simulink model "reference_model"  (R2023a)
settings: Solver=VariableStepAuto  StartTime=0.0  StopTime=200  RelTol=1e-3
values from neighbouring files (symbols this model uses):
  Af = diag ([1/t1, 1/t2, 1/t3])    [init.m]
  Gamma_Matrix = diag(omega.^2)    [init.m]
  Omega_Matrix = diag (2*zeta.*omega)    [init.m]
libraries: eeStairGenerator x3
settings Model: Creator=33769  LastModifiedBy=33769

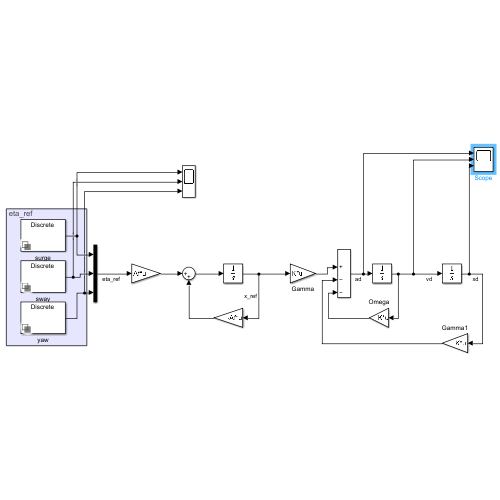
[thumbnail: Simulink's stored preview of the top-level diagram]
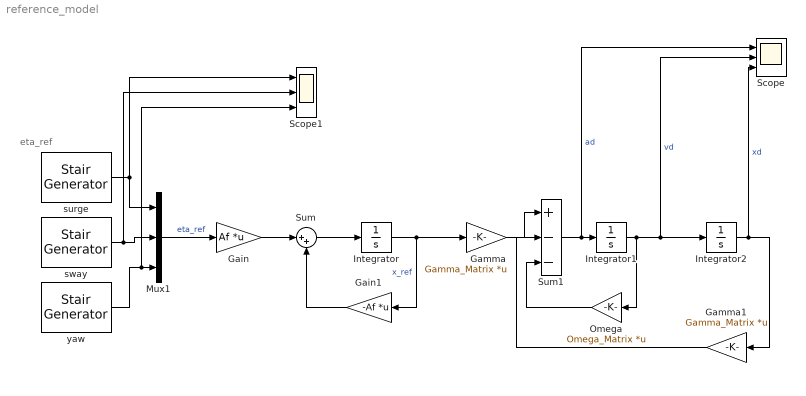
== system reference_model ==
  note: eta_ref
  Gain : Gain  Gain=Af  Multiplication=Matrix(K*u)
  Gain1 : Gain  Gain=-Af  Multiplication=Matrix(K*u)
  Gamma : Gain  Gain=Gamma_Matrix  Multiplication=Matrix(K*u)
  Gamma1 : Gain  Gain=Gamma_Matrix  Multiplication=Matrix(K*u)
  Integrator : Integrator
  Integrator1 : Integrator
  Integrator2 : Integrator
  Mux1 : Mux  Inputs=3
  Omega : Gain  Gain=Omega_Matrix  Multiplication=Matrix(K*u)
  Scope : Scope  NumInputPorts=3
  Scope1 : Scope  NumInputPorts=3
  Sum : Sum  Inputs=|++
  Sum1 : Sum  Inputs=|+--
  surge : eeStairGenerator/Stair Generator  LabelModeActiveChoice=Discrete  TimeInput=[50]  AmplitudeInput=[10]  SampleTime=0.1  RepeatPattern=off  OutDataTypeStr=double
      settings: LibrarySourceBlock=ee_sl_lib/General Control/Stair Generator
  sway : eeStairGenerator/Stair Generator  LabelModeActiveChoice=Discrete  TimeInput=[50]  AmplitudeInput=[10]  SampleTime=0.1  RepeatPattern=off  OutDataTypeStr=double
      settings: LibrarySourceBlock=ee_sl_lib/General Control/Stair Generator
  yaw : eeStairGenerator/Stair Generator  LabelModeActiveChoice=Discrete  TimeInput=[50]  AmplitudeInput=[3*pi/2]  SampleTime=0.1  RepeatPattern=off  OutDataTypeStr=double
      settings: LibrarySourceBlock=ee_sl_lib/General Control/Stair Generator
  wires:
  Gamma1/1 -> Sum1/2
  Integrator1/1 -> Omega/1, Scope/2, Integrator2/1  "vd"
  Sum/1 -> Integrator/1
  Omega/1 -> Sum1/3
  Sum1/1 -> Scope/1, Integrator1/1  "ad"
  Gamma/1 -> Sum1/1
  Integrator2/1 -> Scope/3, Gamma1/1  "xd"
  yaw/1 -> Scope1/3, Mux1/3
  Mux1/1 -> Gain/1  "eta_ref"
  Gain1/1 -> Sum/2
  surge/1 -> Scope1/1, Mux1/1
  Gain/1 -> Sum/1
  Integrator/1 -> Gamma/1, Gain1/1  "x_ref"
  sway/1 -> Scope1/2, Mux1/2
